simulink model "Uebung22_2016a"  (R2016a)
settings: Solver=ode5  SolverMode=SingleTasking  StartTime=0.0  StopTime=10.0  FixedStep=0.1  RelTol=1e-3
values from neighbouring files (symbols this model uses):
  L = 100    [Uebung222.m]
  R = 100    [Uebung222.m]
undefined symbols (not defined in the file or in its folder): LC
settings Model: Creator=Jason  LastModifiedBy=Jason
settings DebuggingCC: SFUnexpectedBacktrackingDiag=error  SFNoUnconditionalDefaultTransitionDiag=error
settings GRTTargetCC: TargetLangStandard=C99 (ISO)  GeneratePreprocessorConditionals=Use local settings
settings ConfigComp: CovMetricSettings=dwe  CovHtmlReporting=off  CovSaveCumulativeToWorkspaceVar=off  CovSaveSingleToWorkspaceVar=off  CovExternalEMLEnable=on

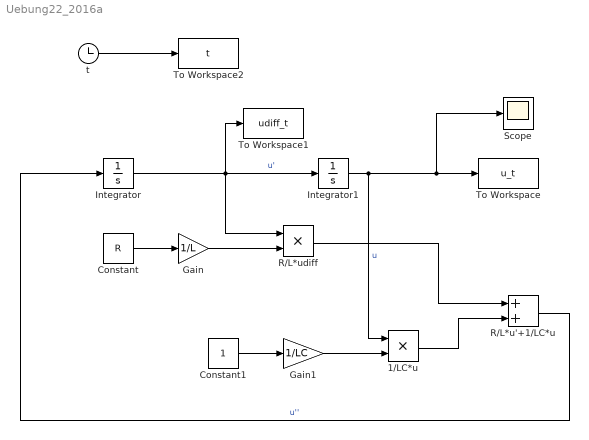
== system Uebung22_2016a ==
  1/LC*u : Product
  Constant : Constant  Value=R
  Constant1 : Constant
  Gain : Gain  Gain=1/L
  Gain1 : Gain  Gain=1/LC
  Integrator : Integrator  InitialCondition=1
  Integrator1 : Integrator  InitialCondition=1
  R/L*u'+1/LC*u : Sum
  R/L*udiff : Product
  Scope : Scope
  To Workspace : ToWorkspace  VariableName=u_t  SampleTime=-1
  To Workspace1 : ToWorkspace  VariableName=udiff_t  SampleTime=-1
  To Workspace2 : ToWorkspace  VariableName=t  SampleTime=-1
  t : Clock
  wires:
  Integrator/1 -> To Workspace1/1, R/L*udiff/1, Integrator1/1  "u'"
  R/L*udiff/1 -> R/L*u'+1/LC*u/1
  t/1 -> To Workspace2/1
  Constant1/1 -> Gain1/1
  Gain1/1 -> 1/LC*u/2
  1/LC*u/1 -> R/L*u'+1/LC*u/2
  Gain/1 -> R/L*udiff/2
  R/L*u'+1/LC*u/1 -> Integrator/1  "u''"
  Integrator1/1 -> Scope/1, To Workspace/1, 1/LC*u/1  "u"
  Constant/1 -> Gain/1
